simulink model "hw_pos_control_pid"  (R2020b)
settings: Solver=ode1  StartTime=0.0  StopTime=60  FixedStep=0.01  RelTol=1e-3  EnableMultiTasking=on
values from neighbouring files (symbols this model uses):
  a = 27.65    [parameter.m]
  b = 17.35    [parameter.m]
  Kd = (2*zeta*wn + lamda_1 -a)/b    (= 0.784244211034)    [parameter.m]
  Ki = (wn^2*lamda_1)/b    (= 0.910165247363)    [parameter.m]
  Kp = (2*zeta*wn*lamda_1 + wn^2)/b    (= 2.91990009415)    [parameter.m]
libraries: arduinolib x12
settings Model: SILPILModeSetting=veronly  ExtModeTrigDuration=2  Creator=ONLY-GOD  LastModifiedBy=ONLY-GOD
settings OptimizationCC: EnhancedBackFolding=on  PassReuseOutputArgsAs=Individual arguments  ZeroExternalMemoryAtStartup=off  ZeroInternalMemoryAtStartup=off  MaxStackSize=64  OptimizeBlockOrder=speed  DifferentSizesBufferReuse=on  OptimizationCustomize=off  EfficientTunableParamExpr=on
settings DebuggingCC: ParameterTunabilityLossMsg=error
settings HardwareCC: ProdBitPerPointer=32  ProdBitPerSizeT=32  ProdBitPerPtrDiffT=32  ProdLargestAtomicInteger=Long  ProdLargestAtomicFloat=Double  ProdWordSize=32  ProdHWDeviceType=ARM Compatible->ARM Cortex
settings SFSimCC: MATLABDynamicMemAlloc=off
settings RTWCC: Description=Embedded Coder  SystemTargetFile=ert.tlc  HardwareBoard=Arduino Due  TemplateMakefile=ert_default_tmf  Toolchain=Arduino ARM  BuildConfiguration=Faster Runs
settings CodeAppCC: ForceParamTrailComments=on  IgnoreCustomStorageClasses=off  OperatorAnnotations=on  SimulinkDataObjDesc=on  SFDataObjDesc=on  InsertBlockDesc=on
settings ERTTargetCC: SupportContinuousTime=on  SupportVariableSizeSignals=on  ExtModeTransport=3  ExtModeStaticAllocSize=24576  ExtModeMexFile=ext_xcp  ExtModeIntrfLevel=Level2 - Open

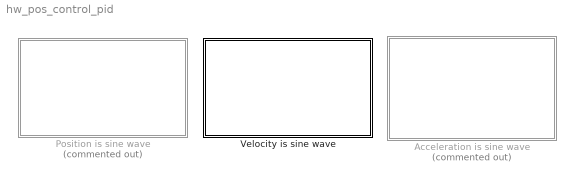
== system hw_pos_control_pid ==
  Acceleration is sine wave : Subsystem  Commented=on
  Position is sine wave : Subsystem  Commented=on
  Velocity is sine wave : Subsystem

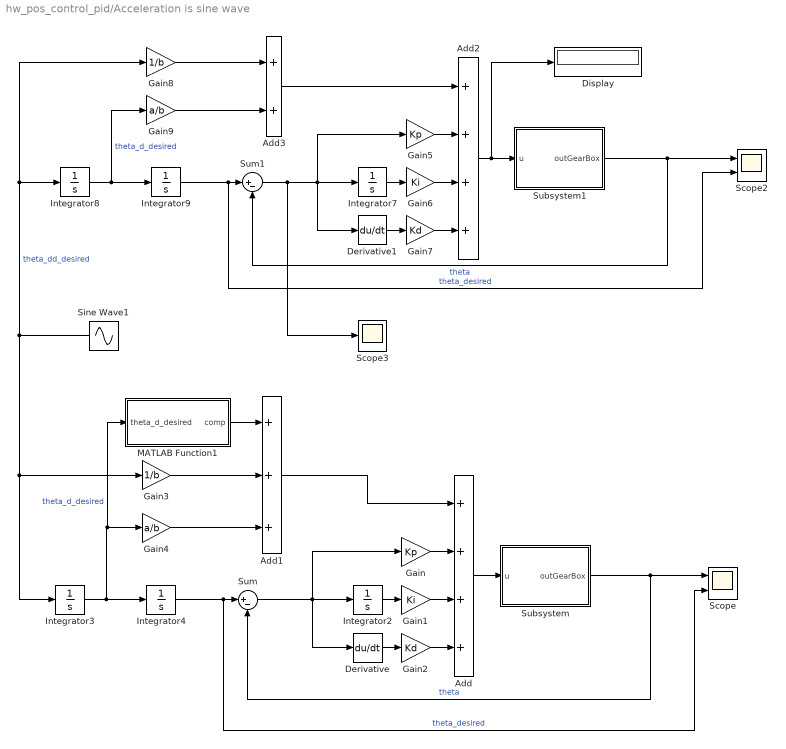
== system hw_pos_control_pid/Acceleration is sine wave ==
  Add : Sum  Inputs=++++
  Add1 : Sum  Inputs=+++
  Add2 : Sum  Inputs=++++
  Add3 : Sum
  Derivative : Derivative
  Derivative1 : Derivative
  Display : Display
  Gain : Gain  Gain=Kp
  Gain1 : Gain  Gain=Ki
  Gain2 : Gain  Gain=Kd
  Gain3 : Gain  Gain=1/b
  Gain4 : Gain  Gain=a/b
  Gain5 : Gain  Gain=Kp
  Gain6 : Gain  Gain=Ki
  Gain7 : Gain  Gain=Kd
  Gain8 : Gain  Gain=1/b
  Gain9 : Gain  Gain=a/b
  Integrator{2..4,7..9} (6 alike) : Integrator
  MATLAB Function1 : MATLAB Function  TreatAsAtomicUnit=on
  Scope : Scope  NumInputPorts=2
  Scope2 : Scope  NumInputPorts=2
  Scope3 : Scope
  Sine Wave1 : Sin  Amplitude=2  Frequency=2*pi*0.1  SampleTime=0
  Subsystem : Subsystem
  Subsystem1 : Subsystem
  Sum : Sum  Inputs=|+-
  Sum1 : Sum  Inputs=|+-
  wires:
  Integrator9/1 -> Sum1/1, Scope2/2  "theta_desired"
  Gain/1 -> Add/2
  Sum/1 -> Derivative/1, Integrator2/1, Gain/1
  Subsystem/1(outGearBox) -> Scope/1, Sum/2  "theta"
  Integrator8/1 -> Integrator9/1, Gain9/1  "theta_d_desired"
  Gain4/1 -> Add1/3
  Derivative/1 -> Gain2/1
  Sine Wave1/1 -> Gain3/1, Integrator3/1, Integrator8/1, Gain8/1  "theta_dd_desired"
  Gain2/1 -> Add/4
  Sum1/1 -> Scope3/1, Gain5/1, Integrator7/1, Derivative1/1
  Integrator3/1 -> MATLAB Function1/1(theta_d_desired), Gain4/1, Integrator4/1  "theta_d_desired"
  Integrator2/1 -> Gain1/1
  Gain1/1 -> Add/3
  Add1/1 -> Add/1
  Integrator4/1 -> Scope/2, Sum/1  "theta_desired"
  Gain6/1 -> Add2/3
  Gain9/1 -> Add3/2
  Subsystem1/1(outGearBox) -> Scope2/1, Sum1/2  "theta"
  Gain3/1 -> Add1/2
  Add2/1 -> Display/1, Subsystem1/1(u)
  Gain5/1 -> Add2/2
  MATLAB Function1/1(comp) -> Add1/1
  Integrator7/1 -> Gain6/1
  Add/1 -> Subsystem/1(u)
  Derivative1/1 -> Gain7/1
  Add3/1 -> Add2/1
  Gain7/1 -> Add2/4
  Gain8/1 -> Add3/1

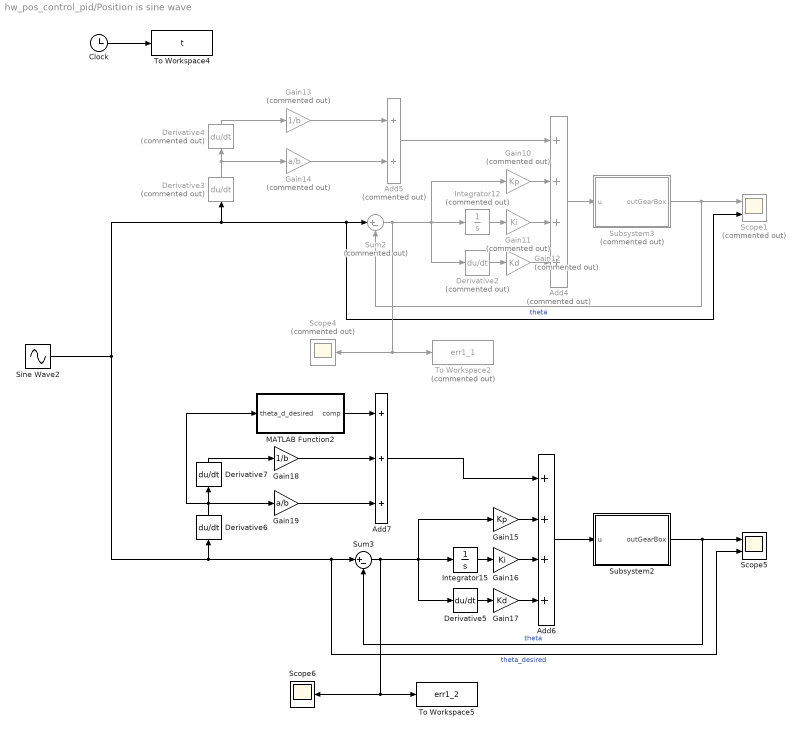
== system hw_pos_control_pid/Position is sine wave ==
  Add4 : Sum  Commented=on  Inputs=++++
  Add5 : Sum  Commented=on
  Add6 : Sum  Inputs=++++
  Add7 : Sum  Inputs=+++
  Clock : Clock
  Derivative2 : Derivative  Commented=on
  Derivative3 : Derivative  Commented=on
  Derivative4 : Derivative  Commented=on
  Derivative5 : Derivative
  Derivative6 : Derivative
  Derivative7 : Derivative
  Gain10 : Gain  Commented=on  Gain=Kp
  Gain11 : Gain  Commented=on  Gain=Ki
  Gain12 : Gain  Commented=on  Gain=Kd
  Gain13 : Gain  Commented=on  Gain=1/b
  Gain14 : Gain  Commented=on  Gain=a/b
  Gain15 : Gain  Gain=Kp
  Gain16 : Gain  Gain=Ki
  Gain17 : Gain  Gain=Kd
  Gain18 : Gain  Gain=1/b
  Gain19 : Gain  Gain=a/b
  Integrator12 : Integrator  Commented=on
  Integrator15 : Integrator
  MATLAB Function2 : MATLAB Function  TreatAsAtomicUnit=on
  Scope1 : Scope  Commented=on  NumInputPorts=2
  Scope4 : Scope  Commented=on
  Scope5 : Scope  NumInputPorts=2
  Scope6 : Scope
  Sine Wave2 : Sin  Amplitude=10  Frequency=2*pi*0.1  SampleTime=0
  Subsystem2 : Subsystem
  Subsystem3 : Subsystem  Commented=on
  Sum2 : Sum  Commented=on  Inputs=|+-
  Sum3 : Sum  Inputs=|+-
  To Workspace2 : ToWorkspace  Commented=on  VariableName=err1_1  SampleTime=-1
      settings: Save2DSignal=2-D array (concatenate along first dimension)
  To Workspace4 : ToWorkspace  VariableName=t  SampleTime=-1
      settings: Save2DSignal=2-D array (concatenate along first dimension)
  To Workspace5 : ToWorkspace  VariableName=err1_2  SampleTime=-1
      settings: Save2DSignal=2-D array (concatenate along first dimension)
  wires:
  Sine Wave2/1 -> Derivative6/1, Sum3/1, Scope5/2, Sum2/1, Scope1/2, Derivative3/1  "theta_desired"
  Subsystem3/1(outGearBox) -> Scope1/1, Sum2/2  "theta"
  Integrator12/1 -> Gain11/1
  Add4/1 -> Subsystem3/1(u)
  Sum2/1 -> To Workspace2/1, Scope4/1, Derivative2/1, Integrator12/1, Gain10/1
  Add6/1 -> Subsystem2/1(u)
  Sum3/1 -> Gain15/1, Integrator15/1, Derivative5/1, To Workspace5/1, Scope6/1
  Gain18/1 -> Add7/2
  Gain10/1 -> Add4/2
  Gain12/1 -> Add4/4
  Derivative6/1 -> Gain19/1, MATLAB Function2/1(theta_d_desired), Derivative7/1
  Derivative3/1 -> Derivative4/1, Gain14/1
  MATLAB Function2/1(comp) -> Add7/1
  Gain13/1 -> Add5/1
  Derivative2/1 -> Gain12/1
  Gain15/1 -> Add6/2
  Clock/1 -> To Workspace4/1
  Subsystem2/1(outGearBox) -> Sum3/2, Scope5/1  "theta"
  Gain19/1 -> Add7/3
  Derivative4/1 -> Gain13/1
  Derivative5/1 -> Gain17/1
  Gain11/1 -> Add4/3
  Gain16/1 -> Add6/3
  Integrator15/1 -> Gain16/1
  Gain17/1 -> Add6/4
  Derivative7/1 -> Gain18/1
  Add7/1 -> Add6/1
  Add5/1 -> Add4/1
  Gain14/1 -> Add5/2

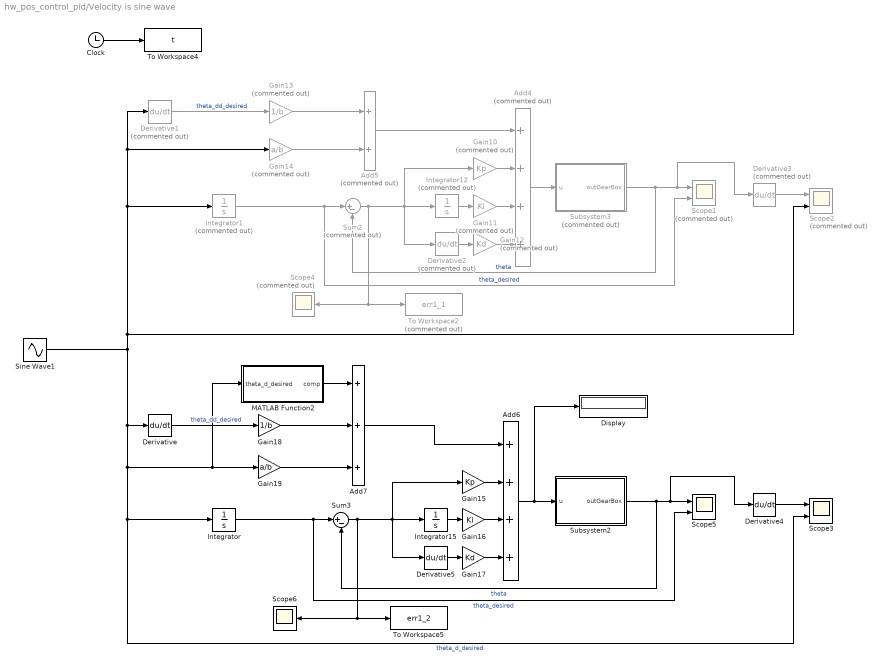
== system hw_pos_control_pid/Velocity is sine wave ==
  Add4 : Sum  Commented=on  Inputs=++++
  Add5 : Sum  Commented=on
  Add6 : Sum  Inputs=++++
  Add7 : Sum  Inputs=+++
  Clock : Clock
  Derivative : Derivative
  Derivative1 : Derivative  Commented=on
  Derivative2 : Derivative  Commented=on
  Derivative3 : Derivative  Commented=on
  Derivative4 : Derivative
  Derivative5 : Derivative
  Display : Display
  Gain10 : Gain  Commented=on  Gain=Kp
  Gain11 : Gain  Commented=on  Gain=Ki
  Gain12 : Gain  Commented=on  Gain=Kd
  Gain13 : Gain  Commented=on  Gain=1/b
  Gain14 : Gain  Commented=on  Gain=a/b
  Gain15 : Gain  Gain=Kp
  Gain16 : Gain  Gain=Ki
  Gain17 : Gain  Gain=Kd
  Gain18 : Gain  Gain=1/b
  Gain19 : Gain  Gain=a/b
  Integrator : Integrator
  Integrator1 : Integrator  Commented=on
  Integrator12 : Integrator  Commented=on
  Integrator15 : Integrator
  MATLAB Function2 : MATLAB Function  TreatAsAtomicUnit=on
  Scope1 : Scope  Commented=on  NumInputPorts=2
  Scope2 : Scope  Commented=on  NumInputPorts=2
  Scope3 : Scope  NumInputPorts=2
  Scope4 : Scope  Commented=on
  Scope5 : Scope  NumInputPorts=2
  Scope6 : Scope
  Sine Wave1 : Sin  Amplitude=10  Frequency=2*pi*0.1  SampleTime=0
  Subsystem2 : Subsystem
  Subsystem3 : Subsystem  Commented=on
  Sum2 : Sum  Commented=on  Inputs=|+-
  Sum3 : Sum  Inputs=|+-
  To Workspace2 : ToWorkspace  Commented=on  VariableName=err1_1  SampleTime=-1
      settings: Save2DSignal=2-D array (concatenate along first dimension)
  To Workspace4 : ToWorkspace  VariableName=t  SampleTime=-1
      settings: Save2DSignal=2-D array (concatenate along first dimension)
  To Workspace5 : ToWorkspace  VariableName=err1_2  SampleTime=-1
      settings: Save2DSignal=2-D array (concatenate along first dimension)
  wires:
  Gain14/1 -> Add5/2
  Add5/1 -> Add4/1
  Add7/1 -> Add6/1
  Gain17/1 -> Add6/4
  Integrator15/1 -> Gain16/1
  Gain16/1 -> Add6/3
  Gain11/1 -> Add4/3
  Derivative5/1 -> Gain17/1
  Gain19/1 -> Add7/3
  Subsystem2/1(outGearBox) -> Derivative4/1, Scope5/1, Sum3/2  "theta"
  Clock/1 -> To Workspace4/1
  Gain15/1 -> Add6/2
  Derivative2/1 -> Gain12/1
  Gain13/1 -> Add5/1
  MATLAB Function2/1(comp) -> Add7/1
  Gain12/1 -> Add4/4
  Gain10/1 -> Add4/2
  Gain18/1 -> Add7/2
  Sum3/1 -> Scope6/1, To Workspace5/1, Derivative5/1, Integrator15/1, Gain15/1
  Add6/1 -> Display/1, Subsystem2/1(u)
  Sum2/1 -> Gain10/1, Integrator12/1, Derivative2/1, Scope4/1, To Workspace2/1
  Add4/1 -> Subsystem3/1(u)
  Integrator12/1 -> Gain11/1
  Subsystem3/1(outGearBox) -> Sum2/2, Derivative3/1, Scope1/1  "theta"
  Sine Wave1/1 -> Gain14/1, Derivative1/1, Integrator1/1, Scope2/2, Derivative/1, Scope3/2, Integrator/1, MATLAB Function2/1(theta_d_desired), Gain19/1  "theta_d_desired"
  Integrator/1 -> Scope5/2, Sum3/1  "theta_desired"
  Derivative/1 -> Gain18/1  "theta_dd_desired"
  Integrator1/1 -> Scope1/2, Sum2/1  "theta_desired"
  Derivative1/1 -> Gain13/1  "theta_dd_desired"
  Derivative3/1 -> Scope2/1
  Derivative4/1 -> Scope3/1

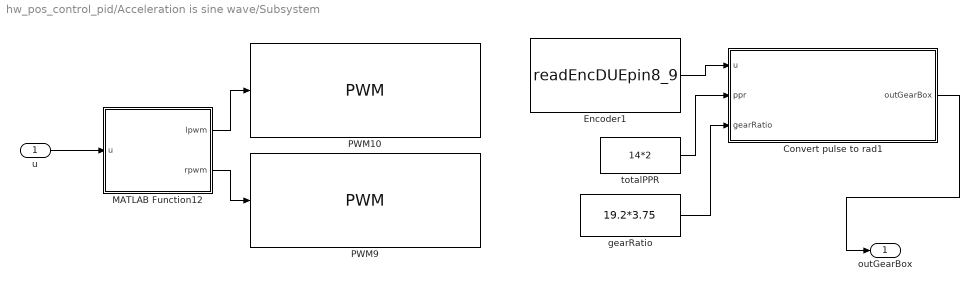
== system hw_pos_control_pid/Acceleration is sine wave/Subsystem ==
  u : Inport
  Convert pulse to rad1 : MATLAB Function  TreatAsAtomicUnit=on
  Encoder1 : S-Function  InitFcn=try, set_param(gcb,'FunctionName','readEncDUEpin8_9'), end  FunctionName=readEncDUEpin8_9  SFunctionModules=readEncDUEpin8_9_wrapper  SFunctionDeploymentMode=off  EnableBusSupport=off  mask(S-Function Builder){}
      mask help: Simulink:masks:SFunctionBuilder_MD
      mask init:
      | val = [[.9  0.75 0.75 1 1 .9 .9 1]',[1 1 0.75 0.75 .9 .9 1 .9]'];try , sys = get_param(gcb,'SfunBuilderFcnName');if isempty(sys), sys = get_param(gcb,'FunctionName'); end,catch, sys = get_param(gcb,'FunctionName'); end
      settings: CopyFcn=set_param(gcbh,'LinkStatus','none')  PreSaveFcn=try, set_param(gcb,'FunctionName','readEncDUEpin8_9'), end  OpenFcn=sfunctionwizard(gcbh)
      mask Display: plot(val(:,1),val(:,2)),disp(sys),port_label('output',1,'count')
  MATLAB Function12 : MATLAB Function  TreatAsAtomicUnit=on
  PWM10 : arduinolib/PWM  pinNumber=7  frequencyType=Default  desiredFrequency=490.2  achievableFrequency=490.2
  PWM9 : arduinolib/PWM  pinNumber=6  frequencyType=Default  desiredFrequency=490.2  achievableFrequency=490.2
  gearRatio : Constant  Value=19.2*3.75
  totalPPR : Constant  Value=14*2
  outGearBox : Outport
  wires:
  Encoder1/1 -> Convert pulse to rad1/1(u)
  MATLAB Function12/1(lpwm) -> PWM10/1
  totalPPR/1 -> Convert pulse to rad1/2(ppr)
  MATLAB Function12/2(rpwm) -> PWM9/1
  gearRatio/1 -> Convert pulse to rad1/3(gearRatio)
  u/1 -> MATLAB Function12/1(u)
  Convert pulse to rad1/1(outGearBox) -> outGearBox/1

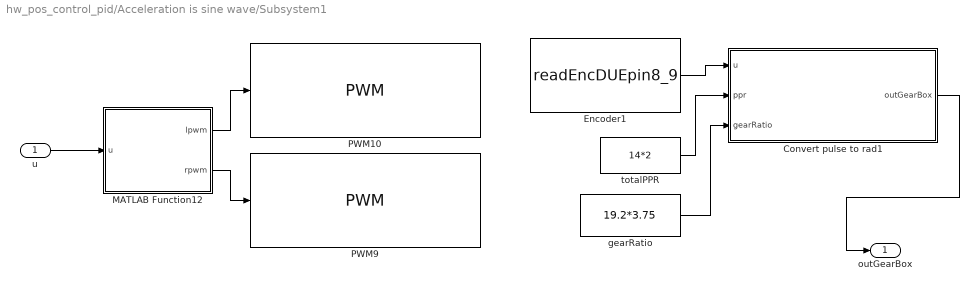
== system hw_pos_control_pid/Acceleration is sine wave/Subsystem1 ==
  u : Inport
  Convert pulse to rad1 : MATLAB Function  TreatAsAtomicUnit=on
  Encoder1 : S-Function  InitFcn=try, set_param(gcb,'FunctionName','readEncDUEpin8_9'), end  FunctionName=readEncDUEpin8_9  SFunctionModules=readEncDUEpin8_9_wrapper  SFunctionDeploymentMode=off  EnableBusSupport=off  mask(S-Function Builder){}
      mask help: Simulink:masks:SFunctionBuilder_MD
      mask init: same as hw_pos_control_pid/Acceleration is sine wave/Subsystem/Encoder1
      settings: CopyFcn=set_param(gcbh,'LinkStatus','none')  PreSaveFcn=try, set_param(gcb,'FunctionName','readEncDUEpin8_9'), end  OpenFcn=sfunctionwizard(gcbh)
      mask Display: plot(val(:,1),val(:,2)),disp(sys),port_label('output',1,'count')
  MATLAB Function12 : MATLAB Function  TreatAsAtomicUnit=on
  PWM10 : arduinolib/PWM  pinNumber=7  frequencyType=Default  desiredFrequency=490.2  achievableFrequency=490.2
  PWM9 : arduinolib/PWM  pinNumber=6  frequencyType=Default  desiredFrequency=490.2  achievableFrequency=490.2
  gearRatio : Constant  Value=19.2*3.75
  totalPPR : Constant  Value=14*2
  outGearBox : Outport
  wires:
  Convert pulse to rad1/1(outGearBox) -> outGearBox/1
  u/1 -> MATLAB Function12/1(u)
  gearRatio/1 -> Convert pulse to rad1/3(gearRatio)
  MATLAB Function12/2(rpwm) -> PWM9/1
  totalPPR/1 -> Convert pulse to rad1/2(ppr)
  MATLAB Function12/1(lpwm) -> PWM10/1
  Encoder1/1 -> Convert pulse to rad1/1(u)

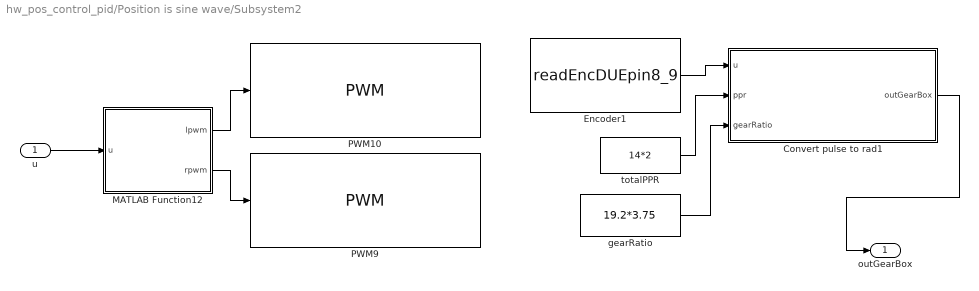
== system hw_pos_control_pid/Position is sine wave/Subsystem2 ==
  u : Inport
  Convert pulse to rad1 : MATLAB Function  TreatAsAtomicUnit=on
  Encoder1 : S-Function  InitFcn=try, set_param(gcb,'FunctionName','readEncDUEpin8_9'), end  FunctionName=readEncDUEpin8_9  SFunctionModules=readEncDUEpin8_9_wrapper  SFunctionDeploymentMode=off  EnableBusSupport=off  mask(S-Function Builder){}
      mask help: Simulink:masks:SFunctionBuilder_MD
      mask init: same as hw_pos_control_pid/Acceleration is sine wave/Subsystem/Encoder1
      settings: CopyFcn=set_param(gcbh,'LinkStatus','none')  PreSaveFcn=try, set_param(gcb,'FunctionName','readEncDUEpin8_9'), end  OpenFcn=sfunctionwizard(gcbh)
      mask Display: plot(val(:,1),val(:,2)),disp(sys),port_label('output',1,'count')
  MATLAB Function12 : MATLAB Function  TreatAsAtomicUnit=on
  PWM10 : arduinolib/PWM  pinNumber=7  frequencyType=Default  desiredFrequency=490.2  achievableFrequency=490.2
  PWM9 : arduinolib/PWM  pinNumber=6  frequencyType=Default  desiredFrequency=490.2  achievableFrequency=490.2
  gearRatio : Constant  Value=19.2*3.75
  totalPPR : Constant  Value=14*2
  outGearBox : Outport
  wires:
  Encoder1/1 -> Convert pulse to rad1/1(u)
  MATLAB Function12/1(lpwm) -> PWM10/1
  totalPPR/1 -> Convert pulse to rad1/2(ppr)
  MATLAB Function12/2(rpwm) -> PWM9/1
  gearRatio/1 -> Convert pulse to rad1/3(gearRatio)
  u/1 -> MATLAB Function12/1(u)
  Convert pulse to rad1/1(outGearBox) -> outGearBox/1

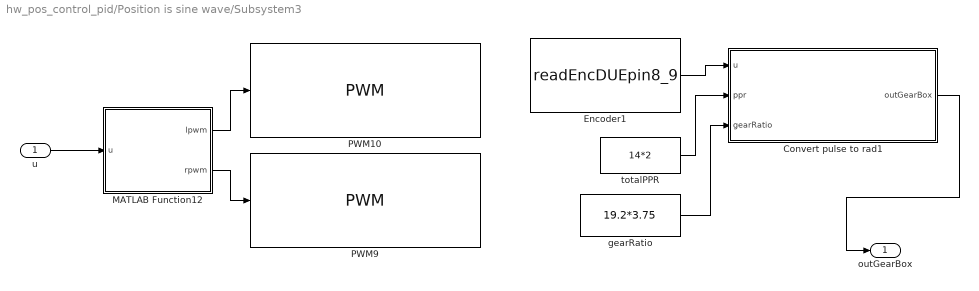
== system hw_pos_control_pid/Position is sine wave/Subsystem3 ==
  u : Inport
  Convert pulse to rad1 : MATLAB Function  TreatAsAtomicUnit=on
  Encoder1 : S-Function  InitFcn=try, set_param(gcb,'FunctionName','readEncDUEpin8_9'), end  FunctionName=readEncDUEpin8_9  SFunctionModules=readEncDUEpin8_9_wrapper  SFunctionDeploymentMode=off  EnableBusSupport=off  mask(S-Function Builder){}
      mask help: Simulink:masks:SFunctionBuilder_MD
      mask init: same as hw_pos_control_pid/Acceleration is sine wave/Subsystem/Encoder1
      settings: CopyFcn=set_param(gcbh,'LinkStatus','none')  PreSaveFcn=try, set_param(gcb,'FunctionName','readEncDUEpin8_9'), end  OpenFcn=sfunctionwizard(gcbh)
      mask Display: plot(val(:,1),val(:,2)),disp(sys),port_label('output',1,'count')
  MATLAB Function12 : MATLAB Function  TreatAsAtomicUnit=on
  PWM10 : arduinolib/PWM  pinNumber=7  frequencyType=Default  desiredFrequency=490.2  achievableFrequency=490.2
  PWM9 : arduinolib/PWM  pinNumber=6  frequencyType=Default  desiredFrequency=490.2  achievableFrequency=490.2
  gearRatio : Constant  Value=19.2*3.75
  totalPPR : Constant  Value=14*2
  outGearBox : Outport
  wires:
  Convert pulse to rad1/1(outGearBox) -> outGearBox/1
  u/1 -> MATLAB Function12/1(u)
  gearRatio/1 -> Convert pulse to rad1/3(gearRatio)
  MATLAB Function12/2(rpwm) -> PWM9/1
  totalPPR/1 -> Convert pulse to rad1/2(ppr)
  MATLAB Function12/1(lpwm) -> PWM10/1
  Encoder1/1 -> Convert pulse to rad1/1(u)

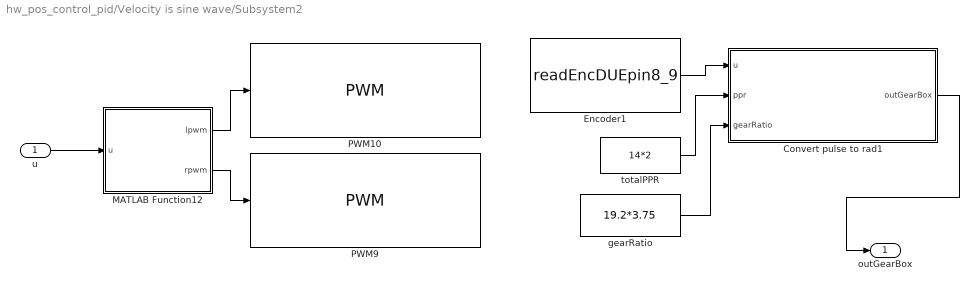
== system hw_pos_control_pid/Velocity is sine wave/Subsystem2 ==
  u : Inport
  Convert pulse to rad1 : MATLAB Function  TreatAsAtomicUnit=on
  Encoder1 : S-Function  InitFcn=try, set_param(gcb,'FunctionName','readEncDUEpin8_9'), end  FunctionName=readEncDUEpin8_9  SFunctionModules=readEncDUEpin8_9_wrapper  SFunctionDeploymentMode=off  EnableBusSupport=off  mask(S-Function Builder){}
      mask help: Simulink:masks:SFunctionBuilder_MD
      mask init: same as hw_pos_control_pid/Acceleration is sine wave/Subsystem/Encoder1
      settings: CopyFcn=set_param(gcbh,'LinkStatus','none')  PreSaveFcn=try, set_param(gcb,'FunctionName','readEncDUEpin8_9'), end  OpenFcn=sfunctionwizard(gcbh)
      mask Display: plot(val(:,1),val(:,2)),disp(sys),port_label('output',1,'count')
  MATLAB Function12 : MATLAB Function  TreatAsAtomicUnit=on
  PWM10 : arduinolib/PWM  pinNumber=7  frequencyType=Default  desiredFrequency=490.2  achievableFrequency=490.2
  PWM9 : arduinolib/PWM  pinNumber=6  frequencyType=Default  desiredFrequency=490.2  achievableFrequency=490.2
  gearRatio : Constant  Value=19.2*3.75
  totalPPR : Constant  Value=14*2
  outGearBox : Outport
  wires:
  Convert pulse to rad1/1(outGearBox) -> outGearBox/1
  u/1 -> MATLAB Function12/1(u)
  gearRatio/1 -> Convert pulse to rad1/3(gearRatio)
  MATLAB Function12/2(rpwm) -> PWM9/1
  totalPPR/1 -> Convert pulse to rad1/2(ppr)
  MATLAB Function12/1(lpwm) -> PWM10/1
  Encoder1/1 -> Convert pulse to rad1/1(u)

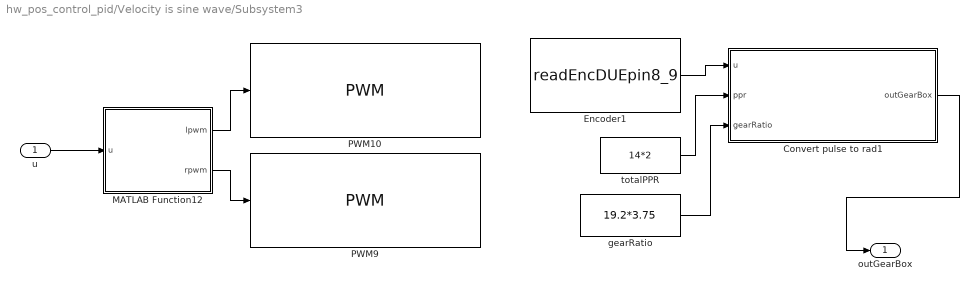
== system hw_pos_control_pid/Velocity is sine wave/Subsystem3 ==
  u : Inport
  Convert pulse to rad1 : MATLAB Function  TreatAsAtomicUnit=on
  Encoder1 : S-Function  InitFcn=try, set_param(gcb,'FunctionName','readEncDUEpin8_9'), end  FunctionName=readEncDUEpin8_9  SFunctionModules=readEncDUEpin8_9_wrapper  SFunctionDeploymentMode=off  EnableBusSupport=off  mask(S-Function Builder){}
      mask help: Simulink:masks:SFunctionBuilder_MD
      mask init: same as hw_pos_control_pid/Acceleration is sine wave/Subsystem/Encoder1
      settings: CopyFcn=set_param(gcbh,'LinkStatus','none')  PreSaveFcn=try, set_param(gcb,'FunctionName','readEncDUEpin8_9'), end  OpenFcn=sfunctionwizard(gcbh)
      mask Display: plot(val(:,1),val(:,2)),disp(sys),port_label('output',1,'count')
  MATLAB Function12 : MATLAB Function  TreatAsAtomicUnit=on
  PWM10 : arduinolib/PWM  pinNumber=7  frequencyType=Default  desiredFrequency=490.2  achievableFrequency=490.2
  PWM9 : arduinolib/PWM  pinNumber=6  frequencyType=Default  desiredFrequency=490.2  achievableFrequency=490.2
  gearRatio : Constant  Value=19.2*3.75
  totalPPR : Constant  Value=14*2
  outGearBox : Outport
  wires:
  Encoder1/1 -> Convert pulse to rad1/1(u)
  MATLAB Function12/1(lpwm) -> PWM10/1
  totalPPR/1 -> Convert pulse to rad1/2(ppr)
  MATLAB Function12/2(rpwm) -> PWM9/1
  gearRatio/1 -> Convert pulse to rad1/3(gearRatio)
  u/1 -> MATLAB Function12/1(u)
  Convert pulse to rad1/1(outGearBox) -> outGearBox/1

== matlab function hw_pos_control_pid/Velocity is sine wave/Subsystem2/MATLAB Function12 ==
  data: u input; lpwm output; rpwm output
function [lpwm,rpwm] = fcn(u)

Vmax = 23.6;
pwm = u*254/Vmax;
if pwm > 0
    lpwm = pwm;
    rpwm = 0;
elseif pwm < 0
    lpwm = 0;
    rpwm = abs(pwm);
else
    lpwm = 0;
    rpwm = 0;
end

== matlab function hw_pos_control_pid/Acceleration is sine wave/Subsystem/Convert pulse to rad1 ==
  settings: updateMethod=DISCRETE
  data: u input; ppr input; gearRatio input; outGearBox output
function outGearBox = fcn(u,ppr,gearRatio)

persistent counter_num over_flag
if(isempty(counter_num)), counter_num = 0;end
if(isempty(over_flag)), over_flag = 0;end
pulse2radian = 2*pi/ppr; % 1 pulse = ?? radian

if(double(u) - counter_num > 40000), over_flag = over_flag-1;
elseif(double(u) - counter_num < -40000), over_flag = over_flag+1;
end

inGearBox = (double(u)+over_flag*(2^32 -1))*pulse2radian; 
outGearBox = inGearBox/gearRatio;
counter_num = double(u) ;

== matlab function hw_pos_control_pid/Velocity is sine wave/Subsystem3/Convert pulse to rad1 ==
  settings: updateMethod=DISCRETE
  data: u input; ppr input; gearRatio input; outGearBox output
function outGearBox = fcn(u,ppr,gearRatio)

persistent counter_num over_flag
if(isempty(counter_num)), counter_num = 0;end
if(isempty(over_flag)), over_flag = 0;end
pulse2radian = 2*pi/ppr; % 1 pulse = ?? radian

if(double(u) - counter_num > 40000), over_flag = over_flag-1;
elseif(double(u) - counter_num < -40000), over_flag = over_flag+1;
end

inGearBox = (double(u)+over_flag*(2^32 -1))*pulse2radian; 
outGearBox = inGearBox/gearRatio;
counter_num = double(u) ;

== matlab function hw_pos_control_pid/Acceleration is sine wave/MATLAB Function1 ==
  settings: updateMethod=DISCRETE
  data: theta_d_desired input; comp output
function comp = fcn(theta_d_desired)

b = 17.35; c = 5.63; %+ 0.3*rand;
comp = c/b*sign(theta_d_desired);

== matlab function hw_pos_control_pid/Velocity is sine wave/Subsystem3/MATLAB Function12 ==
  data: u input; lpwm output; rpwm output
function [lpwm,rpwm] = fcn(u)

Vmax = 23.6;
pwm = u*254/Vmax;
if pwm > 0
    lpwm = pwm;
    rpwm = 0;
elseif pwm < 0
    lpwm = 0;
    rpwm = abs(pwm);
else
    lpwm = 0;
    rpwm = 0;
end

== matlab function hw_pos_control_pid/Acceleration is sine wave/Subsystem1/Convert pulse to rad1 ==
  settings: updateMethod=DISCRETE
  data: u input; ppr input; gearRatio input; outGearBox output
function outGearBox = fcn(u,ppr,gearRatio)

persistent counter_num over_flag
if(isempty(counter_num)), counter_num = 0;end
if(isempty(over_flag)), over_flag = 0;end
pulse2radian = 2*pi/ppr; % 1 pulse = ?? radian

if(double(u) - counter_num > 40000), over_flag = over_flag-1;
elseif(double(u) - counter_num < -40000), over_flag = over_flag+1;
end

inGearBox = (double(u)+over_flag*(2^32 -1))*pulse2radian; 
outGearBox = inGearBox/gearRatio;
counter_num = double(u) ;

== matlab function hw_pos_control_pid/Acceleration is sine wave/Subsystem1/MATLAB Function12 ==
  data: u input; lpwm output; rpwm output
function [lpwm,rpwm] = fcn(u)

Vmax = 23.6;
pwm = u*254/Vmax;
if pwm > 0
    lpwm = pwm;
    rpwm = 0;
elseif pwm < 0
    lpwm = 0;
    rpwm = abs(pwm);
else
    lpwm = 0;
    rpwm = 0;
end

== matlab function hw_pos_control_pid/Velocity is sine wave/MATLAB Function2 ==
  settings: updateMethod=DISCRETE
  data: theta_d_desired input; comp output
function comp = fcn(theta_d_desired)

b = 17.35; c = 5.63; %+ 0.3*rand;
comp = c/b*sign(theta_d_desired);

== matlab function hw_pos_control_pid/Acceleration is sine wave/Subsystem/MATLAB Function12 ==
  data: u input; lpwm output; rpwm output
function [lpwm,rpwm] = fcn(u)

Vmax = 23.6;
pwm = u*254/Vmax;
if pwm > 0
    lpwm = pwm;
    rpwm = 0;
elseif pwm < 0
    lpwm = 0;
    rpwm = abs(pwm);
else
    lpwm = 0;
    rpwm = 0;
end

== matlab function hw_pos_control_pid/Position is sine wave/MATLAB Function2 ==
  settings: updateMethod=DISCRETE
  data: theta_d_desired input; comp output
function comp = fcn(theta_d_desired)

b = 17.35; c = 5.63; %+ 0.3*rand;
comp = c/b*sign(theta_d_desired);

== matlab function hw_pos_control_pid/Velocity is sine wave/Subsystem2/Convert pulse to rad1 ==
  settings: updateMethod=DISCRETE
  data: u input; ppr input; gearRatio input; outGearBox output
function outGearBox = fcn(u,ppr,gearRatio)

persistent counter_num over_flag
if(isempty(counter_num)), counter_num = 0;end
if(isempty(over_flag)), over_flag = 0;end
pulse2radian = 2*pi/ppr; % 1 pulse = ?? radian

if(double(u) - counter_num > 40000), over_flag = over_flag-1;
elseif(double(u) - counter_num < -40000), over_flag = over_flag+1;
end

inGearBox = (double(u)+over_flag*(2^32 -1))*pulse2radian; 
outGearBox = inGearBox/gearRatio;
counter_num = double(u) ;

== matlab function hw_pos_control_pid/Position is sine wave/Subsystem2/Convert pulse to rad1 ==
  settings: updateMethod=DISCRETE
  data: u input; ppr input; gearRatio input; outGearBox output
function outGearBox = fcn(u,ppr,gearRatio)

persistent counter_num over_flag
if(isempty(counter_num)), counter_num = 0;end
if(isempty(over_flag)), over_flag = 0;end
pulse2radian = 2*pi/ppr; % 1 pulse = ?? radian

if(double(u) - counter_num > 40000), over_flag = over_flag-1;
elseif(double(u) - counter_num < -40000), over_flag = over_flag+1;
end

inGearBox = (double(u)+over_flag*(2^32 -1))*pulse2radian; 
outGearBox = inGearBox/gearRatio;
counter_num = double(u) ;

== matlab function hw_pos_control_pid/Position is sine wave/Subsystem2/MATLAB Function12 ==
  data: u input; lpwm output; rpwm output
function [lpwm,rpwm] = fcn(u)

Vmax = 23.6;
pwm = u*254/Vmax;
if pwm > 0
    lpwm = pwm;
    rpwm = 0;
elseif pwm < 0
    lpwm = 0;
    rpwm = abs(pwm);
else
    lpwm = 0;
    rpwm = 0;
end

== matlab function hw_pos_control_pid/Position is sine wave/Subsystem3/Convert pulse to rad1 ==
  settings: updateMethod=DISCRETE
  data: u input; ppr input; gearRatio input; outGearBox output
function outGearBox = fcn(u,ppr,gearRatio)

persistent counter_num over_flag
if(isempty(counter_num)), counter_num = 0;end
if(isempty(over_flag)), over_flag = 0;end
pulse2radian = 2*pi/ppr; % 1 pulse = ?? radian

if(double(u) - counter_num > 40000), over_flag = over_flag-1;
elseif(double(u) - counter_num < -40000), over_flag = over_flag+1;
end

inGearBox = (double(u)+over_flag*(2^32 -1))*pulse2radian; 
outGearBox = inGearBox/gearRatio;
counter_num = double(u) ;

== matlab function hw_pos_control_pid/Position is sine wave/Subsystem3/MATLAB Function12 ==
  data: u input; lpwm output; rpwm output
function [lpwm,rpwm] = fcn(u)

Vmax = 23.6;
pwm = u*254/Vmax;
if pwm > 0
    lpwm = pwm;
    rpwm = 0;
elseif pwm < 0
    lpwm = 0;
    rpwm = abs(pwm);
else
    lpwm = 0;
    rpwm = 0;
end
